simulink model "model_comp_19b"  (R2019b)
settings: Solver=ode45  StartTime=0.0  StopTime=100  RelTol=1e-3  EnableMultiTasking=on
values from neighbouring files (symbols this model uses):
  KDspd = 0    [time_validation.m]
  KIspd = 0    [time_validation.m]
  KPspd = 20    [time_validation.m]
  PARSa = [ ... (first row only)    [Q_ART_par.m]
  PARSu = zeros(Nu,5)    [Q_ART_par.m]
  TOTALMASS = sum (M,'all')    [Q_ART_par.m]
  v_ref = vconst    (= 5.55555555556)    [time_validation.m]
undefined symbols (not defined in the file or in its folder): axle_rate_limit, BRAKE, brake_lag, brake_rate, DRIVE, Lspd, Nspd, RW, Tb, Tst, Uspd
libraries: CarMaker4SL x72, simulink x2, TruckMaker4SL x1
(part 2 of 3)

== system model_comp_19b/truckmaker model/TruckMaker/IPG Vehicle/CarAndTrailer/Steering ==
  note: When replacing the entire steering system,
      | be sure to disable the IPG steering model by using the steering
      | model 'Model Manager off' in the vehicle GUI.
  Sync_In : Inport
  VhclCtrl.Steering : Inport  Port=2
  Bus Creator1 : BusCreator  Inputs=16
  Bus Creator2 : BusCreator  Inputs=5
  Demux : Demux  Outputs=21
      settings: DisplayOption=none
  Steering : S-Function  FunctionName=TM_Sfun  Parameters='Steering'  SFunctionDeploymentMode=off  EnableBusSupport=off
  Terminator : Terminator
  Sync_Out : Outport
  Steer.IF : Outport  Port=2
  wires:
  Demux/21 -> Bus Creator2/5  "Steering IF R Inert"
  Demux/20 -> Bus Creator2/4  "Steering IF R Frc"
  Demux/19 -> Bus Creator2/3  "Steering IF L Inert"
  Demux/18 -> Bus Creator2/2  "Steering IF L Frc"
  Demux/17 -> Bus Creator2/1  "Steering IF SteerByTrq"
  Demux/16 -> Bus Creator1/16  "Steering IF R iSteer2q"
  Demux/15 -> Bus Creator1/15  "Steering IF R qpp"
  Demux/14 -> Bus Creator1/14  "Steering IF R qp"
  Demux/13 -> Bus Creator1/13  "Steering IF R q"
  Demux/12 -> Bus Creator1/12  "Steering IF L iSteer2q"
  Demux/11 -> Bus Creator1/11  "Steering IF L qpp"
  Demux/10 -> Bus Creator1/10  "Steering IF L qp"
  Demux/9 -> Bus Creator1/9  "Steering IF L q"
  Demux/8 -> Bus Creator1/8  "Steering IF AssistTrqPin"
  Demux/7 -> Bus Creator1/7  "Steering IF AssistTrqCol"
  Demux/6 -> Bus Creator1/6  "Steering IF AssistFrc"
  Demux/5 -> Bus Creator1/5  "Steering IF TrqStatic"
  Demux/4 -> Bus Creator1/4  "Steering IF Trq"
  Demux/3 -> Bus Creator1/3  "Steering IF AngAcc"
  Demux/2 -> Bus Creator1/2  "Steering IF AngVel"
  Demux/1 -> Bus Creator1/1  "Steering IF Ang"
  Bus Creator1/1 -> Steer.IF/1
  Bus Creator2/1 -> Terminator/1  "Steer IF (in)"
  Sync_In/1 -> Steering/1
  Steering/1 -> Sync_Out/1
  VhclCtrl.Steering/1 -> Steering/2
  Steering/2 -> Demux/1

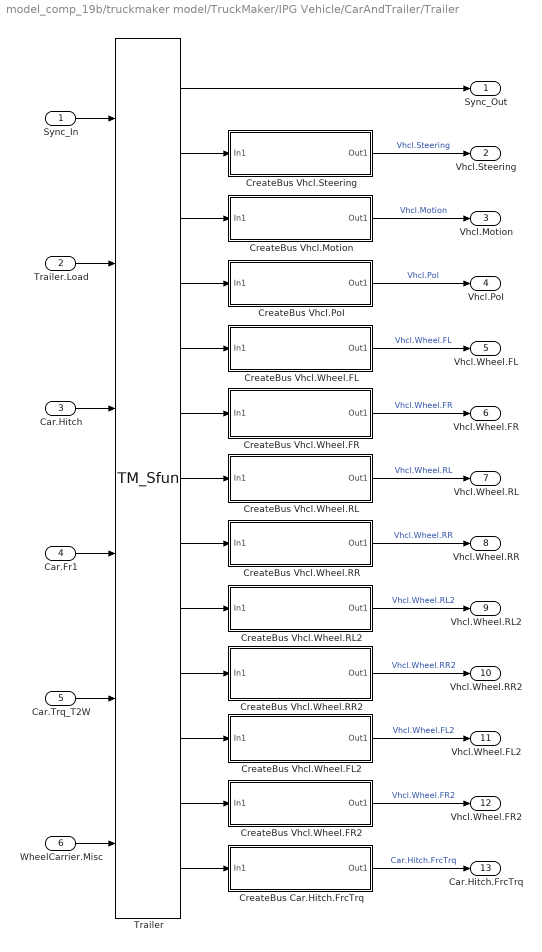
== system model_comp_19b/truckmaker model/TruckMaker/IPG Vehicle/CarAndTrailer/Trailer ==
  Sync_In : Inport
  Trailer.Load : Inport  Port=2
  Car.Hitch : Inport  Port=3
  Car.Fr1 : Inport  Port=4
  Car.Trq_T2W : Inport  Port=5
  WheelCarrier.Misc : Inport  Port=6
  CreateBus Car.Hitch.FrcTrq : Subsystem
  CreateBus Vhcl.Motion : Subsystem
  CreateBus Vhcl.PoI : Subsystem
  CreateBus Vhcl.Steering : Subsystem
  CreateBus Vhcl.Wheel.FL : Subsystem
  CreateBus Vhcl.Wheel.FL2 : Subsystem
  CreateBus Vhcl.Wheel.FR : Subsystem
  CreateBus Vhcl.Wheel.FR2 : Subsystem
  CreateBus Vhcl.Wheel.RL : Subsystem
  CreateBus Vhcl.Wheel.RL2 : Subsystem
  CreateBus Vhcl.Wheel.RR : Subsystem
  CreateBus Vhcl.Wheel.RR2 : Subsystem
  Trailer : S-Function  FunctionName=TM_Sfun  Parameters='Trailer'  SFunctionDeploymentMode=off  EnableBusSupport=off
  Sync_Out : Outport
  Vhcl.Steering : Outport  Port=2
  Vhcl.Motion : Outport  Port=3
  Vhcl.PoI : Outport  Port=4
  Vhcl.Wheel.FL : Outport  Port=5
  Vhcl.Wheel.FR : Outport  Port=6
  Vhcl.Wheel.RL : Outport  Port=7
  Vhcl.Wheel.RR : Outport  Port=8
  Vhcl.Wheel.RL2 : Outport  Port=9
  Vhcl.Wheel.RR2 : Outport  Port=10
  Vhcl.Wheel.FL2 : Outport  Port=11
  Vhcl.Wheel.FR2 : Outport  Port=12
  Car.Hitch.FrcTrq : Outport  Port=13
  wires:
  CreateBus Vhcl.Wheel.RL2/1(Out1) -> Vhcl.Wheel.RL2/1  "Vhcl.Wheel.RL2"
  CreateBus Vhcl.Wheel.RR2/1(Out1) -> Vhcl.Wheel.RR2/1  "Vhcl.Wheel.RR2"
  CreateBus Vhcl.Wheel.FL2/1(Out1) -> Vhcl.Wheel.FL2/1  "Vhcl.Wheel.FL2"
  CreateBus Vhcl.Wheel.FR2/1(Out1) -> Vhcl.Wheel.FR2/1  "Vhcl.Wheel.FR2"
  Trailer/12 -> CreateBus Vhcl.Wheel.FR2/1(In1)
  Trailer/11 -> CreateBus Vhcl.Wheel.FL2/1(In1)
  Trailer/10 -> CreateBus Vhcl.Wheel.RR2/1(In1)
  Trailer/9 -> CreateBus Vhcl.Wheel.RL2/1(In1)
  CreateBus Vhcl.Wheel.FL/1(Out1) -> Vhcl.Wheel.FL/1  "Vhcl.Wheel.FL"
  CreateBus Vhcl.Wheel.FR/1(Out1) -> Vhcl.Wheel.FR/1  "Vhcl.Wheel.FR"
  CreateBus Vhcl.Wheel.RL/1(Out1) -> Vhcl.Wheel.RL/1  "Vhcl.Wheel.RL"
  CreateBus Vhcl.Wheel.RR/1(Out1) -> Vhcl.Wheel.RR/1  "Vhcl.Wheel.RR"
  Trailer/8 -> CreateBus Vhcl.Wheel.RR/1(In1)
  Trailer/7 -> CreateBus Vhcl.Wheel.RL/1(In1)
  Trailer/6 -> CreateBus Vhcl.Wheel.FR/1(In1)
  Trailer/5 -> CreateBus Vhcl.Wheel.FL/1(In1)
  Trailer/13 -> CreateBus Car.Hitch.FrcTrq/1(In1)
  Trailer/2 -> CreateBus Vhcl.Steering/1(In1)
  CreateBus Vhcl.Steering/1(Out1) -> Vhcl.Steering/1  "Vhcl.Steering"
  Trailer/3 -> CreateBus Vhcl.Motion/1(In1)
  Trailer/4 -> CreateBus Vhcl.PoI/1(In1)
  CreateBus Vhcl.PoI/1(Out1) -> Vhcl.PoI/1  "Vhcl.PoI"
  CreateBus Vhcl.Motion/1(Out1) -> Vhcl.Motion/1  "Vhcl.Motion"
  Car.Trq_T2W/1 -> Trailer/5
  WheelCarrier.Misc/1 -> Trailer/6
  CreateBus Car.Hitch.FrcTrq/1(Out1) -> Car.Hitch.FrcTrq/1  "Car.Hitch.FrcTrq"
  Car.Fr1/1 -> Trailer/4
  Car.Hitch/1 -> Trailer/3
  Trailer.Load/1 -> Trailer/2
  Trailer/1 -> Sync_Out/1
  Sync_In/1 -> Trailer/1

== system model_comp_19b/truckmaker model/TruckMaker/IPG Vehicle/AFGc/brake and drive controller1/1&2 axle ==
  drive torque 1&2 : Inport
  Constant2 : Constant  Value=0
  Gain{,1..3} (4 alike) : Gain  Gain=-1
  Gain4 : Gain  Commented=through  Gain=-1
  To Workspace : ToWorkspace  VariableName=drive_torque1  SampleTime=-1
  Write CM Dict : CarMaker4SL/Write CM Dict  xname=PT.WFL.Trq_Drive  xsync=off
  Write CM Dict1 : CarMaker4SL/Write CM Dict  xname=PT.WFR.Trq_Drive  xsync=off
  Write CM Dict2 : CarMaker4SL/Write CM Dict  xname=PT.WRL.Trq_Drive  xsync=off
  Write CM Dict3 : CarMaker4SL/Write CM Dict  xname=PT.WRR.Trq_Drive  xsync=off
  Write CM Dict4 : CarMaker4SL/Write CM Dict  xname=PT.WFL.Trq_Supp2WC  xsync=off
  Write CM Dict5 : CarMaker4SL/Write CM Dict  xname=PT.WFR.Trq_Supp2WC  xsync=off
  Write CM Dict6 : CarMaker4SL/Write CM Dict  xname=PT.WRL.Trq_Supp2WC  xsync=off
  Write CM Dict7 : CarMaker4SL/Write CM Dict  xname=PT.WRR.Trq_Supp2WC  xsync=off
  Write CM Dict8 : CarMaker4SL/Write CM Dict  xname=PT.Trq_Supp2Bdy1B.y  xsync=off
  Write CM Dict9 : CarMaker4SL/Write CM Dict  xname=PT.Trq_Supp2Bdy1.y  xsync=off
  wires:
  Gain/1 -> Write CM Dict4/1
  Gain1/1 -> Write CM Dict5/1
  Gain2/1 -> Write CM Dict6/1
  Constant2/1 -> Write CM Dict8/1, Write CM Dict9/1
  drive torque 1&2/1 -> Gain4/1
  Gain3/1 -> Write CM Dict7/1
  Gain4/1 -> Gain/1, Write CM Dict/1, Gain1/1, Write CM Dict1/1, Write CM Dict2/1, Gain2/1, Gain3/1, Write CM Dict3/1, To Workspace/1

== system model_comp_19b/truckmaker model/TruckMaker/IPG Vehicle/AFGc/brake and drive controller1/7&8 axle ==
  drive torque 7&8 : Inport
  Gain4 : Gain  Commented=through  Gain=-1
  Terminator : Terminator  Commented=on
  To Workspace : ToWorkspace  VariableName=drive_torque7_8  SampleTime=-1
  Write CM Dict1 : CarMaker4SL/Write CM Dict  xname=Tr2.Trq_Ext2WhlML  xsync=off
  Write CM Dict2 : CarMaker4SL/Write CM Dict  xname=Tr2.Trq_Ext2WhlRL  xsync=off
  Write CM Dict3 : CarMaker4SL/Write CM Dict  xname=Tr2.Trq_Ext2WhlRR  xsync=off
  Write CM Dict4 : CarMaker4SL/Write CM Dict  xname=Tr2.Trq_Ext2WhlMR  xsync=off
  wires:
  drive torque 7&8/1 -> Gain4/1, To Workspace/1
  Gain4/1 -> Write CM Dict1/1, Write CM Dict4/1, Write CM Dict3/1, Write CM Dict2/1

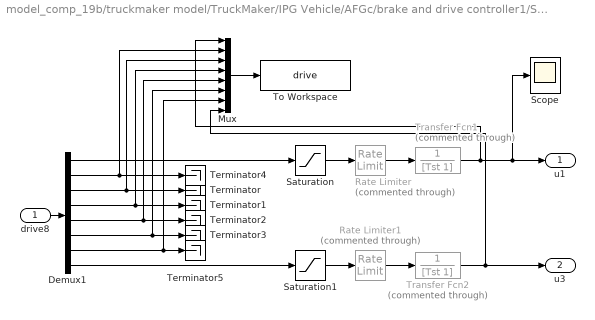
== system model_comp_19b/truckmaker model/TruckMaker/IPG Vehicle/AFGc/brake and drive controller1/Subsystem ==
  drive8 : Inport
  Demux1 : Demux  Outputs=8
  Mux : Mux  Inputs=8
  Rate Limiter : RateLimiter  Commented=through  RisingSlewLimit=500  FallingSlewLimit=-500  SampleTimeMode=inherited
  Rate Limiter1 : RateLimiter  Commented=through  RisingSlewLimit=500  FallingSlewLimit=-500  SampleTimeMode=inherited
  Saturation : Saturate  UpperLimit=1500  LowerLimit=0
  Saturation1 : Saturate  UpperLimit=1500  LowerLimit=0
  Scope : Scope
  Terminator{,1..5} (6 alike) : Terminator
  To Workspace : ToWorkspace  VariableName=drive  SampleTime=-1
  Transfer Fcn1 : TransferFcn  Commented=through  Denominator=[Tst 1]
  Transfer Fcn2 : TransferFcn  Commented=through  Denominator=[Tst 1]
  u1 : Outport
  u3 : Outport  Port=2
  wires:
  Demux1/3 -> Terminator/1, Mux/3
  Demux1/8 -> Saturation1/1
  Demux1/4 -> Terminator1/1, Mux/4
  drive8/1 -> Demux1/1
  Demux1/7 -> Terminator5/1, Mux/7
  Transfer Fcn2/1 -> Mux/8, u3/1
  Demux1/2 -> Mux/2, Terminator4/1
  Saturation1/1 -> Rate Limiter1/1
  Transfer Fcn1/1 -> Mux/1, Scope/1, u1/1
  Saturation/1 -> Rate Limiter/1
  Demux1/5 -> Terminator2/1, Mux/5
  Mux/1 -> To Workspace/1
  Demux1/6 -> Terminator3/1, Mux/6
  Demux1/1 -> Saturation/1
  Rate Limiter1/1 -> Transfer Fcn2/1
  Rate Limiter/1 -> Transfer Fcn1/1

== system model_comp_19b/truckmaker model/TruckMaker/IPG Vehicle/AFGc/brake and drive controller1/brakes ==
  note: torque reverses if wheel goes backwards
  brake torque command : Inport
  wheel speed : Inport  Port=2
  Memory : Memory
  Product : Product
  Rate Limiter : RateLimiter  RisingSlewLimit=brake_rate  FallingSlewLimit=-brake_rate  SampleTimeMode=inherited
  Sign : Signum
  Transport Delay : TransportDelay  Commented=on  DelayTime=brake_lag
  first_order_lags : Subsystem  Commented=on
  Out1 : Outport  VectorParamsAs1DForOutWhenUnconnected=off
  wires:
  Sign/1 -> Product/2
  Product/1 -> Out1/1
  Memory/1 -> Sign/1
  wheel speed/1 -> Memory/1
  Rate Limiter/1 -> Product/1
  Transport Delay/1 -> first_order_lags/1(In1)
  brake torque command/1 -> Rate Limiter/1

== system model_comp_19b/truckmaker model/TruckMaker/IPG Vehicle/AFGc/brake and drive controller1/brakes1 ==
  note: torque reverses if wheel goes backwards
  brake torque command : Inport
  wheel speed : Inport  Port=2
  Memory : Memory
  Product : Product
  Rate Limiter : RateLimiter  RisingSlewLimit=brake_rate  FallingSlewLimit=-brake_rate  SampleTimeMode=inherited
  Sign : Signum
  Transport Delay : TransportDelay  Commented=on  DelayTime=brake_lag
  first_order_lags : Subsystem  Commented=on
  Out1 : Outport  VectorParamsAs1DForOutWhenUnconnected=off
  wires:
  Sign/1 -> Product/2
  Product/1 -> Out1/1
  Memory/1 -> Sign/1
  wheel speed/1 -> Memory/1
  Rate Limiter/1 -> Product/1
  Transport Delay/1 -> first_order_lags/1(In1)
  brake torque command/1 -> Rate Limiter/1

== system model_comp_19b/truckmaker model/TruckMaker/IPG Vehicle/AFGc/brake and drive controller1/brakes2 ==
  note: torque reverses if wheel goes backwards
  brake torque command : Inport
  wheel speed : Inport  Port=2
  Memory : Memory
  Product : Product
  Rate Limiter : RateLimiter  RisingSlewLimit=brake_rate  FallingSlewLimit=-brake_rate  SampleTimeMode=inherited
  Sign : Signum
  Transport Delay : TransportDelay  Commented=on  DelayTime=brake_lag
  first_order_lags : Subsystem  Commented=on
  Out1 : Outport  VectorParamsAs1DForOutWhenUnconnected=off
  wires:
  Sign/1 -> Product/2
  Product/1 -> Out1/1
  Memory/1 -> Sign/1
  wheel speed/1 -> Memory/1
  Rate Limiter/1 -> Product/1
  Transport Delay/1 -> first_order_lags/1(In1)
  brake torque command/1 -> Rate Limiter/1

== system model_comp_19b/truckmaker model/TruckMaker/IPG Vehicle/AFGc/brake and drive controller1/passive torque distrubution ==
  note: convert to torque
  accel command : Inport
  BRAKE : Gain  Gain=BRAKE
  Constant : Constant  Value=0
  FWD : Gain  Gain=DRIVE
  Switch : Switch  Criteria=u2 > Threshold
  Switch1 : Switch  Criteria=u2 > Threshold
  "convert to 'total torque at the wheels\"" : Gain  Gain=TOTALMASS*RW  Multiplication=Matrix(K*u)
  drive torques : Outport  VectorParamsAs1DForOutWhenUnconnected=off
  brake torques : Outport  Port=2  VectorParamsAs1DForOutWhenUnconnected=off
  wires:
  accel command/1 -> "convert to 'total torque at the wheels\""/1
  Constant/1 -> Switch/3, Switch1/1
  Switch/1 -> FWD/1
  FWD/1 -> drive torques/1
  Switch1/1 -> BRAKE/1
  BRAKE/1 -> brake torques/1
  "convert to 'total torque at the wheels\""/1 -> Switch1/3, Switch1/2, Switch/1, Switch/2

== system model_comp_19b/truckmaker model/TruckMaker/IPG Vehicle/AFGc/brake and drive controller1/wheel speeds ==
  Mux1 : Mux  Inputs=3
  Read CM Dict1 : CarMaker4SL/Read CM Dict  xname=Car.WheelSpd_RL2  xsync=off  xstime=Continuous
  Read CM Dict10 : CarMaker4SL/Read CM Dict  xname=Car.WheelSpd_RL  xsync=off  xstime=Continuous
  Read CM Dict8 : CarMaker4SL/Read CM Dict  xname=Car.WheelSpd_FL  xsync=off  xstime=Continuous
  wheel speeds : Outport  VectorParamsAs1DForOutWhenUnconnected=off
  wires:
  Mux1/1 -> wheel speeds/1
  Read CM Dict1/1 -> Mux1/3
  Read CM Dict8/1 -> Mux1/1
  Read CM Dict10/1 -> Mux1/2

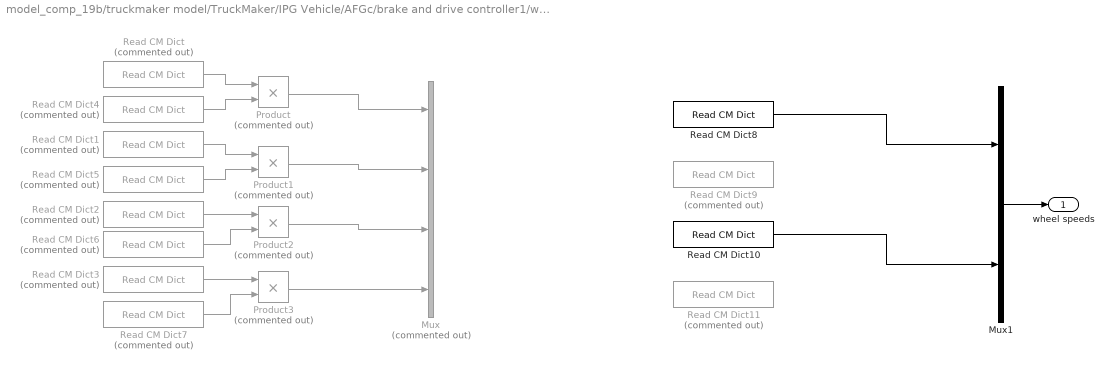
== system model_comp_19b/truckmaker model/TruckMaker/IPG Vehicle/AFGc/brake and drive controller1/wheel speeds1 ==
  Mux : Mux  Commented=on
  Mux1 : Mux  Inputs=2
  Product{,1..3} (4 alike) : Product  Commented=on
  Read CM Dict : CarMaker4SL/Read CM Dict  Commented=on  xname=Car.WheelSpd_FL  xsync=off  xstime=Continuous
  Read CM Dict1 : CarMaker4SL/Read CM Dict  Commented=on  xname=Car.WheelSpd_FR  xsync=off  xstime=Continuous
  Read CM Dict10 : CarMaker4SL/Read CM Dict  xname=Tr.WheelSpd_RL  xsync=off  xstime=Continuous
  Read CM Dict11 : CarMaker4SL/Read CM Dict  Commented=on  xname=Car.WheelSpd_RR  xsync=off  xstime=Continuous
  Read CM Dict2 : CarMaker4SL/Read CM Dict  Commented=on  xname=Car.WheelSpd_RL  xsync=off  xstime=Continuous
  Read CM Dict3 : CarMaker4SL/Read CM Dict  Commented=on  xname=Car.WheelSpd_RR  xsync=off  xstime=Continuous
  Read CM Dict4 : CarMaker4SL/Read CM Dict  Commented=on  xname=Car.WFL.Radius  xsync=off  xstime=Continuous
  Read CM Dict5 : CarMaker4SL/Read CM Dict  Commented=on  xname=Car.WFR.Radius  xsync=off  xstime=Continuous
  Read CM Dict6 : CarMaker4SL/Read CM Dict  Commented=on  xname=Car.WRL.Radius  xsync=off  xstime=Continuous
  Read CM Dict7 : CarMaker4SL/Read CM Dict  Commented=on  xname=Car.WRR.Radius  xsync=off  xstime=Continuous
  Read CM Dict8 : CarMaker4SL/Read CM Dict  xname=Tr.WheelSpd_FL  xsync=off  xstime=Continuous
  Read CM Dict9 : CarMaker4SL/Read CM Dict  Commented=on  xname=Car.WheelSpd_FR  xsync=off  xstime=Continuous
  wheel speeds : Outport  VectorParamsAs1DForOutWhenUnconnected=off
  wires:
  Read CM Dict/1 -> Product/1
  Read CM Dict4/1 -> Product/2
  Read CM Dict1/1 -> Product1/1
  Read CM Dict5/1 -> Product1/2
  Read CM Dict2/1 -> Product2/1
  Read CM Dict6/1 -> Product2/2
  Read CM Dict3/1 -> Product3/1
  Read CM Dict7/1 -> Product3/2
  Product/1 -> Mux/1
  Product1/1 -> Mux/2
  Product2/1 -> Mux/3
  Product3/1 -> Mux/4
  Mux1/1 -> wheel speeds/1
  Read CM Dict8/1 -> Mux1/1
  Read CM Dict10/1 -> Mux1/2

== system model_comp_19b/truckmaker model/TruckMaker/IPG Vehicle/AFGc/brake and drive controller1/wheel speeds2 ==
  Mux1 : Mux  Inputs=3
  Read CM Dict1 : CarMaker4SL/Read CM Dict  xname=Car.WheelSpd_RL  xsync=off  xstime=Continuous
  Read CM Dict10 : CarMaker4SL/Read CM Dict  xname=Car.WheelSpd_RL2  xsync=off  xstime=Continuous
  Read CM Dict8 : CarMaker4SL/Read CM Dict  xname=Car.WheelSpd_FL  xsync=off  xstime=Continuous
  wheel speeds : Outport  VectorParamsAs1DForOutWhenUnconnected=off
  wires:
  Mux1/1 -> wheel speeds/1
  Read CM Dict8/1 -> Mux1/1
  Read CM Dict10/1 -> Mux1/3
  Read CM Dict1/1 -> Mux1/2

== system model_comp_19b/truckmaker model/TruckMaker/IPG Vehicle/AFGc/q&qd builder/build q ==
  Read CM Dict : CarMaker4SL/Read CM Dict  xname=Tr.Yaw  xsync=off  xstime=Continuous
  Read CM Dict1 : CarMaker4SL/Read CM Dict  xname=Car.Yaw  xsync=off  xstime=Continuous
  Read CM Dict2 : CarMaker4SL/Read CM Dict  xname=Tr2.Yaw  xsync=off  xstime=Continuous
  Read CM Dict3 : CarMaker4SL/Read CM Dict  xname=Car.Fr1.tx  xsync=off  xstime=Continuous
  Read CM Dict5 : CarMaker4SL/Read CM Dict  xname=Car.Fr1.ty  xsync=off  xstime=Continuous
  generate q : MATLAB Function  TreatAsAtomicUnit=on
  q : Outport
  wires:
  Read CM Dict3/1 -> generate q/1(FR1x)
  Read CM Dict2/1 -> generate q/5(u3_yaw)
  Read CM Dict/1 -> generate q/4(u2_yaw)
  Read CM Dict1/1 -> generate q/3(u1_yaw)
  generate q/1(q) -> q/1
  Read CM Dict5/1 -> generate q/2(FR1y)

== system model_comp_19b/truckmaker model/TruckMaker/IPG Vehicle/AFGc/q&qd builder/build qd ==
  Read CM Dict1 : CarMaker4SL/Read CM Dict  xname=Car.Yaw  xsync=off  xstime=Continuous
  Read CM Dict2 : CarMaker4SL/Read CM Dict  xname=Tr.YawVel  xsync=off  xstime=Continuous
  Read CM Dict30 : CarMaker4SL/Read CM Dict  xname=Car.YawRate  xsync=off  xstime=Continuous
  Read CM Dict31 : CarMaker4SL/Read CM Dict  xname=Car.Fr1.vx  xsync=off  xstime=Continuous
  Read CM Dict32 : CarMaker4SL/Read CM Dict  xname=Car.Fr1.vy  xsync=off  xstime=Continuous
  Read CM Dict6 : CarMaker4SL/Read CM Dict  xname=Tr2.YawVel  xsync=off  xstime=Continuous
  generate qd : MATLAB Function  TreatAsAtomicUnit=on
  qd : Outport
  wires:
  Read CM Dict31/1 -> generate qd/1(vxFR1)
  Read CM Dict32/1 -> generate qd/2(vyFR1)
  Read CM Dict30/1 -> generate qd/3(u1_yaw_rate)
  Read CM Dict2/1 -> generate qd/4(u2_yaw_rate)
  Read CM Dict6/1 -> generate qd/5(u3_yaw_rate)
  Read CM Dict1/1 -> generate qd/6(u1_yaw_angle)
  generate qd/1(q_d) -> qd/1

== system model_comp_19b/truckmaker model/TruckMaker/IPG Vehicle/CarAndTrailer/CarAndTrailerUpd/CreateBus Brake.IF.In ==
  In : Inport
  BusCreator : BusCreator  Inputs=17
  Demux : Demux  Outputs=17
      settings: DisplayOption=none
  Out : Outport
  wires:
  Demux/17 -> BusCreator/17  "Brake IF Trq_Reg FR2"
  Demux/16 -> BusCreator/16  "Brake IF Trq_Reg FL2"
  Demux/15 -> BusCreator/15  "Brake IF Trq_Reg RR2"
  Demux/14 -> BusCreator/14  "Brake IF Trq_Reg RL2"
  Demux/13 -> BusCreator/13  "Brake IF Trq_Reg RR"
  Demux/12 -> BusCreator/12  "Brake IF Trq_Reg RL"
  Demux/11 -> BusCreator/11  "Brake IF Trq_Reg FR"
  Demux/10 -> BusCreator/10  "Brake IF Trq_Reg FL"
  Demux/9 -> BusCreator/9  "Brake IF Trq_Reg_max FR2"
  Demux/8 -> BusCreator/8  "Brake IF Trq_Reg_max FL2"
  Demux/7 -> BusCreator/7  "Brake IF Trq_Reg_max RR2"
  Demux/6 -> BusCreator/6  "Brake IF Trq_Reg_max RL2"
  Demux/5 -> BusCreator/5  "Brake IF Trq_Reg_max RR"
  Demux/4 -> BusCreator/4  "Brake IF Trq_Reg_max RL"
  Demux/3 -> BusCreator/3  "Brake IF Trq_Reg_max FR"
  Demux/2 -> BusCreator/2  "Brake IF Trq_Reg_max FL"
  Demux/1 -> BusCreator/1  "Brake IF T_env"
  BusCreator/1 -> Out/1
  In/1 -> Demux/1

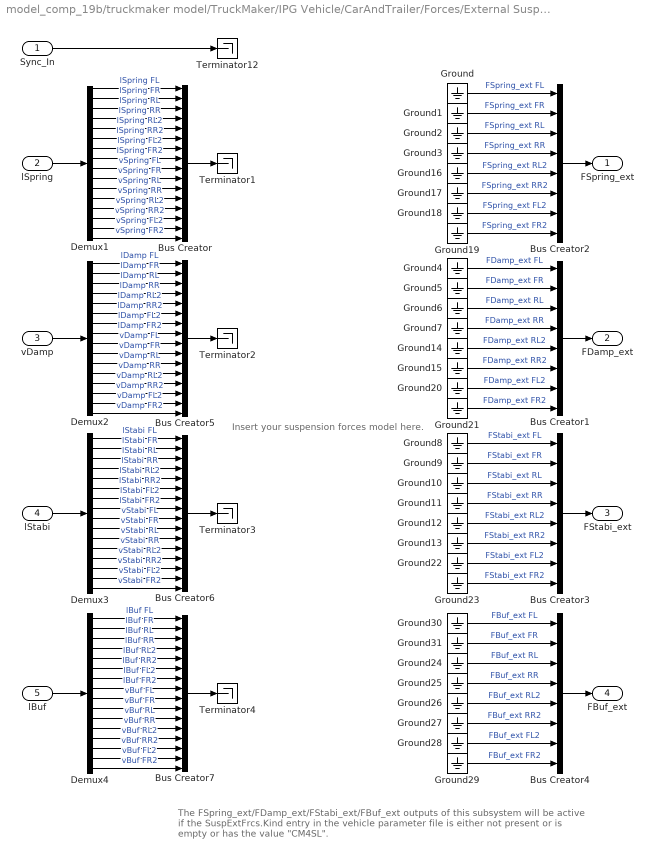
== system model_comp_19b/truckmaker model/TruckMaker/IPG Vehicle/CarAndTrailer/Forces/External Suspension Forces ==
  note: The FSpring_ext/FDamp_ext/FStabi_ext/FBuf_ext outputs of this subsystem will be
      | active if the SuspExtFrcs.Kind entry in the vehicle parameter file
      | is either not present or is empty or has the value "CM4SL".
  note: Insert your suspension forces model here.
  Sync_In : Inport
  lSpring : Inport  Port=2
  vDamp : Inport  Port=3
  lStabi : Inport  Port=4
  lBuf : Inport  Port=5
  Bus Creator{,5..7} (4 alike) : BusCreator  Inputs=16
  Bus Creator{1..4} (4 alike) : BusCreator  Inputs=8
  Demux{1..4} (4 alike) : Demux  Outputs=16
      settings: DisplayOption=none
  Ground{,1..31} (32 alike) : Ground
  Terminator{1..4,12} (5 alike) : Terminator
  FSpring_ext : Outport
  FDamp_ext : Outport  Port=2
  FStabi_ext : Outport  Port=3
  FBuf_ext : Outport  Port=4
  wires:
  Demux3/10 -> Bus Creator6/10  "vStabi FR"
  Demux4/16 -> Bus Creator7/16  "vBuf FR2"
  Demux4/15 -> Bus Creator7/15  "vBuf FL2"
  Demux4/14 -> Bus Creator7/14  "vBuf RR2"
  Demux4/13 -> Bus Creator7/13  "vBuf RL2"
  Demux4/12 -> Bus Creator7/12  "vBuf RR"
  Demux4/11 -> Bus Creator7/11  "vBuf RL"
  Demux4/10 -> Bus Creator7/10  "vBuf FR"
  Demux4/9 -> Bus Creator7/9  "vBuf FL"
  Demux3/16 -> Bus Creator6/16  "vStabi FR2"
  Demux3/15 -> Bus Creator6/15  "vStabi FL2"
  Demux3/14 -> Bus Creator6/14  "vStabi RR2"
  Demux3/13 -> Bus Creator6/13  "vStabi RL2"
  Demux3/12 -> Bus Creator6/12  "vStabi RR"
  Demux3/11 -> Bus Creator6/11  "vStabi RL"
  Demux3/9 -> Bus Creator6/9  "vStabi FL"
  Bus Creator6/1 -> Terminator3/1
  Bus Creator7/1 -> Terminator4/1
  Bus Creator5/1 -> Terminator2/1
  Bus Creator/1 -> Terminator1/1
  Demux2/16 -> Bus Creator5/16  "vDamp FR2"
  Demux2/15 -> Bus Creator5/15  "vDamp FL2"
  Demux2/14 -> Bus Creator5/14  "vDamp RR2"
  Demux2/13 -> Bus Creator5/13  "vDamp RL2"
  Demux2/12 -> Bus Creator5/12  "vDamp RR"
  Demux2/11 -> Bus Creator5/11  "vDamp RL"
  Demux2/10 -> Bus Creator5/10  "vDamp FR"
  Demux2/9 -> Bus Creator5/9  "vDamp FL"
  Demux1/16 -> Bus Creator/16  "vSpring FR2"
  Demux1/15 -> Bus Creator/15  "vSpring FL2"
  Demux1/14 -> Bus Creator/14  "vSpring RR2"
  Demux1/13 -> Bus Creator/13  "vSpring RL2"
  Demux1/12 -> Bus Creator/12  "vSpring RR"
  Demux1/11 -> Bus Creator/11  "vSpring RL"
  Demux1/10 -> Bus Creator/10  "vSpring FR"
  Demux1/9 -> Bus Creator/9  "vSpring FL"
  Demux3/7 -> Bus Creator6/7  "lStabi FL2"
  Demux3/8 -> Bus Creator6/8  "lStabi FR2"
  Ground22/1 -> Bus Creator3/7  "FStabi_ext FL2"
  Ground23/1 -> Bus Creator3/8  "FStabi_ext FR2"
  Demux2/7 -> Bus Creator5/7  "lDamp FL2"
  Demux2/8 -> Bus Creator5/8  "lDamp FR2"
  Ground20/1 -> Bus Creator1/7  "FDamp_ext FL2"
  Ground21/1 -> Bus Creator1/8  "FDamp_ext FR2"
  Ground18/1 -> Bus Creator2/7  "FSpring_ext FL2"
  Ground19/1 -> Bus Creator2/8  "FSpring_ext FR2"
  Demux1/7 -> Bus Creator/7  "lSpring FL2"
  Demux1/8 -> Bus Creator/8  "lSpring FR2"
  Sync_In/1 -> Terminator12/1
  lSpring/1 -> Demux1/1
  vDamp/1 -> Demux2/1
  lStabi/1 -> Demux3/1
  Demux3/1 -> Bus Creator6/1  "lStabi FL"
  Demux3/2 -> Bus Creator6/2  "lStabi FR"
  Demux3/3 -> Bus Creator6/3  "lStabi RL"
  Demux3/4 -> Bus Creator6/4  "lStabi RR"
  Demux1/1 -> Bus Creator/1  "lSpring FL"
  Demux1/2 -> Bus Creator/2  "lSpring FR"
  Demux1/3 -> Bus Creator/3  "lSpring RL"
  Demux1/4 -> Bus Creator/4  "lSpring RR"
  Demux2/1 -> Bus Creator5/1  "lDamp FL"
  Demux2/2 -> Bus Creator5/2  "lDamp FR"
  Demux2/3 -> Bus Creator5/3  "lDamp RL"
  Demux2/4 -> Bus Creator5/4  "lDamp RR"
  Bus Creator2/1 -> FSpring_ext/1
  Ground/1 -> Bus Creator2/1  "FSpring_ext FL"
  Ground1/1 -> Bus Creator2/2  "FSpring_ext FR"
  Ground2/1 -> Bus Creator2/3  "FSpring_ext RL"
  Ground3/1 -> Bus Creator2/4  "FSpring_ext RR"
  Ground4/1 -> Bus Creator1/1  "FDamp_ext FL"
  Ground5/1 -> Bus Creator1/2  "FDamp_ext FR"
  Ground6/1 -> Bus Creator1/3  "FDamp_ext RL"
  Ground7/1 -> Bus Creator1/4  "FDamp_ext RR"
  Bus Creator1/1 -> FDamp_ext/1
  Ground8/1 -> Bus Creator3/1  "FStabi_ext FL"
  Ground9/1 -> Bus Creator3/2  "FStabi_ext FR"
  Ground10/1 -> Bus Creator3/3  "FStabi_ext RL"
  Ground11/1 -> Bus Creator3/4  "FStabi_ext RR"
  Bus Creator3/1 -> FStabi_ext/1
  Demux3/5 -> Bus Creator6/5  "lStabi RL2"
  Demux3/6 -> Bus Creator6/6  "lStabi RR2"
  Ground12/1 -> Bus Creator3/5  "FStabi_ext RL2"
  Ground13/1 -> Bus Creator3/6  "FStabi_ext RR2"
  Demux2/5 -> Bus Creator5/5  "lDamp RL2"
  Demux2/6 -> Bus Creator5/6  "lDamp RR2"
  Ground14/1 -> Bus Creator1/5  "FDamp_ext RL2"
  Ground15/1 -> Bus Creator1/6  "FDamp_ext RR2"
  Demux1/5 -> Bus Creator/5  "lSpring RL2"
  Demux1/6 -> Bus Creator/6  "lSpring RR2"
  Ground16/1 -> Bus Creator2/5  "FSpring_ext RL2"
  Ground17/1 -> Bus Creator2/6  "FSpring_ext RR2"
  Demux4/7 -> Bus Creator7/7  "lBuf FL2"
  Demux4/8 -> Bus Creator7/8  "lBuf FR2"
  Ground28/1 -> Bus Creator4/7  "FBuf_ext FL2"
  Ground29/1 -> Bus Creator4/8  "FBuf_ext FR2"
  lBuf/1 -> Demux4/1
  Demux4/1 -> Bus Creator7/1  "lBuf FL"
  Demux4/2 -> Bus Creator7/2  "lBuf FR"
  Demux4/3 -> Bus Creator7/3  "lBuf RL"
  Demux4/4 -> Bus Creator7/4  "lBuf RR"
  Ground30/1 -> Bus Creator4/1  "FBuf_ext FL"
  Ground31/1 -> Bus Creator4/2  "FBuf_ext FR"
  Ground24/1 -> Bus Creator4/3  "FBuf_ext RL"
  Ground25/1 -> Bus Creator4/4  "FBuf_ext RR"
  Bus Creator4/1 -> FBuf_ext/1
  Demux4/5 -> Bus Creator7/5  "lBuf RL2"
  Demux4/6 -> Bus Creator7/6  "lBuf RR2"
  Ground26/1 -> Bus Creator4/5  "FBuf_ext RL2"
  Ground27/1 -> Bus Creator4/6  "FBuf_ext RR2"

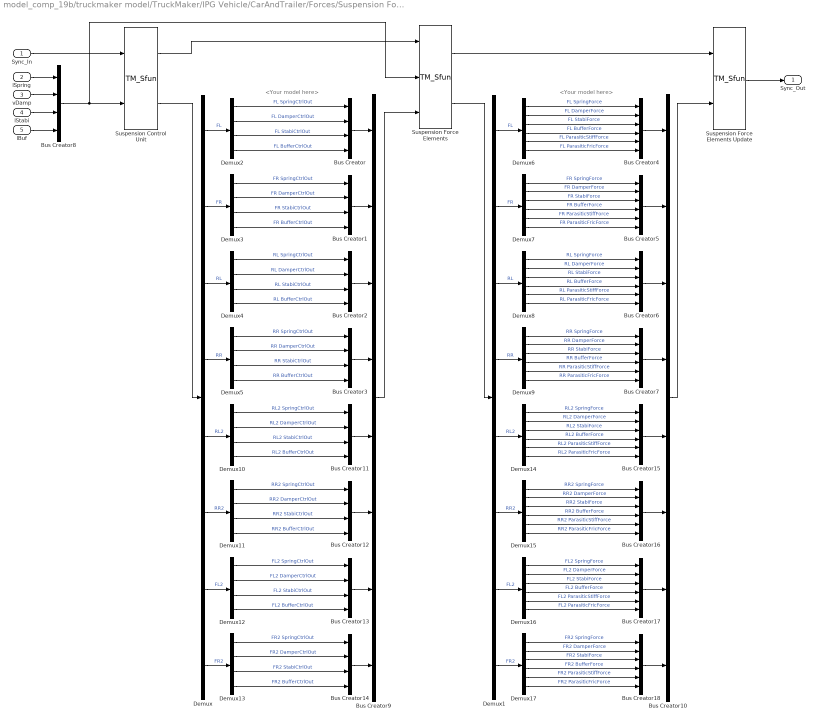
== system model_comp_19b/truckmaker model/TruckMaker/IPG Vehicle/CarAndTrailer/Forces/Suspension Forces ==
  note: <Your model here>
  note: <Your model here>
  Sync_In : Inport
  lSpring : Inport  Port=2
  vDamp : Inport  Port=3
  lStabi : Inport  Port=4
  lBuf : Inport  Port=5
  Bus Creator{,1..3,8,11..14} (9 alike) : BusCreator  Inputs=4
  Bus Creator10 : BusCreator  Inputs=8
  Bus Creator{4..7,15..18} (8 alike) : BusCreator  Inputs=6
  Bus Creator9 : BusCreator  Inputs=8
  Demux : Demux  Outputs=8
  Demux1 : Demux  Outputs=8
  Demux{2..5,10..13} (8 alike) : Demux
  Demux{6..9,14..17} (8 alike) : Demux  Outputs=6
  Suspension Control Unit : S-Function  FunctionName=TM_Sfun  Parameters='ForcesSuspControl'  SFunctionDeploymentMode=off  EnableBusSupport=off
  Suspension Force Elements : S-Function  FunctionName=TM_Sfun  Parameters='ForcesSusp'  SFunctionDeploymentMode=off  EnableBusSupport=off
  Suspension Force Elements Update : S-Function  FunctionName=TM_Sfun  Parameters='ForcesSuspUpd'  SFunctionDeploymentMode=off  EnableBusSupport=off
  Sync_Out : Outport
  wires:
  vDamp/1 -> Bus Creator8/2
  lStabi/1 -> Bus Creator8/3
  lBuf/1 -> Bus Creator8/4
  lSpring/1 -> Bus Creator8/1
  Bus Creator8/1 -> Suspension Control Unit/2, Suspension Force Elements/2
  Sync_In/1 -> Suspension Control Unit/1
  Suspension Control Unit/1 -> Suspension Force Elements/1
  Suspension Force Elements/1 -> Suspension Force Elements Update/1
  Suspension Force Elements Update/1 -> Sync_Out/1
  Bus Creator4/1 -> Bus Creator10/1
  Bus Creator5/1 -> Bus Creator10/2
  Bus Creator6/1 -> Bus Creator10/3
  Bus Creator7/1 -> Bus Creator10/4
  Demux6/1 -> Bus Creator4/1  "FL SpringForce"
  Demux9/1 -> Bus Creator7/1  "RR SpringForce"
  Demux9/2 -> Bus Creator7/2  "RR DamperForce"
  Demux9/3 -> Bus Creator7/3  "RR StabiForce"
  Demux9/4 -> Bus Creator7/4  "RR BufferForce"
  Demux9/5 -> Bus Creator7/5  "RR ParasiticStiffForce"
  Demux9/6 -> Bus Creator7/6  "RR ParasiticFricForce"
  Demux8/1 -> Bus Creator6/1  "RL SpringForce"
  Demux8/2 -> Bus Creator6/2  "RL DamperForce"
  Demux8/4 -> Bus Creator6/4  "RL BufferForce"
  Demux8/5 -> Bus Creator6/5  "RL ParasiticStiffForce"
  Demux8/6 -> Bus Creator6/6  "RL ParasiticFricForce"
  Demux8/3 -> Bus Creator6/3  "RL StabiForce"
  Demux7/1 -> Bus Creator5/1  "FR SpringForce"
  Demux7/2 -> Bus Creator5/2  "FR DamperForce"
  Demux7/3 -> Bus Creator5/3  "FR StabiForce"
  Demux7/4 -> Bus Creator5/4  "FR BufferForce"
  Demux7/5 -> Bus Creator5/5  "FR ParasiticStiffForce"
  Demux7/6 -> Bus Creator5/6  "FR ParasiticFricForce"
  Demux6/2 -> Bus Creator4/2  "FL DamperForce"
  Demux6/3 -> Bus Creator4/3  "FL StabiForce"
  Demux6/4 -> Bus Creator4/4  "FL BufferForce"
  Demux6/5 -> Bus Creator4/5  "FL ParasiticStiffForce"
  Demux6/6 -> Bus Creator4/6  "FL ParasiticFricForce"
  Bus Creator10/1 -> Suspension Force Elements Update/2
  Demux/1 -> Demux2/1  "FL"
  Bus Creator1/1 -> Bus Creator9/2
  Demux/2 -> Demux3/1  "FR"
  Bus Creator2/1 -> Bus Creator9/3
  Demux/3 -> Demux4/1  "RL"
  Bus Creator3/1 -> Bus Creator9/4
  Demux2/1 -> Bus Creator/1  "FL SpringCtrlOut"
  Demux/4 -> Demux5/1  "RR"
  Demux5/1 -> Bus Creator3/1  "RR SpringCtrlOut"
  Demux5/2 -> Bus Creator3/2  "RR DamperCtrlOut"
  Demux5/3 -> Bus Creator3/3  "RR StabiCtrlOut"
  Demux5/4 -> Bus Creator3/4  "RR BufferCtrlOut"
  Demux4/1 -> Bus Creator2/1  "RL SpringCtrlOut"
  Demux4/2 -> Bus Creator2/2  "RL DamperCtrlOut"
  Demux4/4 -> Bus Creator2/4  "RL BufferCtrlOut"
  Demux4/3 -> Bus Creator2/3  "RL StabiCtrlOut"
  Demux3/1 -> Bus Creator1/1  "FR SpringCtrlOut"
  Demux3/2 -> Bus Creator1/2  "FR DamperCtrlOut"
  Demux3/3 -> Bus Creator1/3  "FR StabiCtrlOut"
  Demux3/4 -> Bus Creator1/4  "FR BufferCtrlOut"
  Demux2/2 -> Bus Creator/2  "FL DamperCtrlOut"
  Demux2/3 -> Bus Creator/3  "FL StabiCtrlOut"
  Demux2/4 -> Bus Creator/4  "FL BufferCtrlOut"
  Suspension Control Unit/2 -> Demux/1
  Bus Creator9/1 -> Suspension Force Elements/3
  Bus Creator/1 -> Bus Creator9/1
  Suspension Force Elements/2 -> Demux1/1
  Demux1/1 -> Demux6/1  "FL"
  Demux1/2 -> Demux7/1  "FR"
  Demux1/3 -> Demux8/1  "RL"
  Demux1/4 -> Demux9/1  "RR"
  Demux/5 -> Demux10/1  "RL2"
  Bus Creator12/1 -> Bus Creator9/6
  Demux/6 -> Demux11/1  "RR2"
  Bus Creator13/1 -> Bus Creator9/7
  Demux/7 -> Demux12/1  "FL2"
  Bus Creator14/1 -> Bus Creator9/8
  Demux10/1 -> Bus Creator11/1  "RL2 SpringCtrlOut"
  Demux/8 -> Demux13/1  "FR2"
  Demux13/1 -> Bus Creator14/1  "FR2 SpringCtrlOut"
  Demux13/2 -> Bus Creator14/2  "FR2 DamperCtrlOut"
  Demux13/3 -> Bus Creator14/3  "FR2 StabiCtrlOut"
  Demux13/4 -> Bus Creator14/4  "FR2 BufferCtrlOut"
  Demux12/1 -> Bus Creator13/1  "FL2 SpringCtrlOut"
  Demux12/2 -> Bus Creator13/2  "FL2 DamperCtrlOut"
  Demux12/4 -> Bus Creator13/4  "FL2 BufferCtrlOut"
  Demux12/3 -> Bus Creator13/3  "FL2 StabiCtrlOut"
  Demux11/1 -> Bus Creator12/1  "RR2 SpringCtrlOut"
  Demux11/2 -> Bus Creator12/2  "RR2 DamperCtrlOut"
  Demux11/3 -> Bus Creator12/3  "RR2 StabiCtrlOut"
  Demux11/4 -> Bus Creator12/4  "RR2 BufferCtrlOut"
  Demux10/2 -> Bus Creator11/2  "RL2 DamperCtrlOut"
  Demux10/3 -> Bus Creator11/3  "RL2 StabiCtrlOut"
  Demux10/4 -> Bus Creator11/4  "RL2 BufferCtrlOut"
  Bus Creator11/1 -> Bus Creator9/5
  Bus Creator15/1 -> Bus Creator10/5
  Bus Creator16/1 -> Bus Creator10/6
  Bus Creator17/1 -> Bus Creator10/7
  Bus Creator18/1 -> Bus Creator10/8
  Demux14/1 -> Bus Creator15/1  "RL2 SpringForce"
  Demux17/1 -> Bus Creator18/1  "FR2 SpringForce"
  Demux17/2 -> Bus Creator18/2  "FR2 DamperForce"
  Demux17/3 -> Bus Creator18/3  "FR2 StabiForce"
  Demux17/4 -> Bus Creator18/4  "FR2 BufferForce"
  Demux17/5 -> Bus Creator18/5  "FR2 ParasiticStiffForce"
  Demux17/6 -> Bus Creator18/6  "FR2 ParasiticFricForce"
  Demux16/1 -> Bus Creator17/1  "FL2 SpringForce"
  Demux16/2 -> Bus Creator17/2  "FL2 DamperForce"
  Demux16/4 -> Bus Creator17/4  "FL2 BufferForce"
  Demux16/5 -> Bus Creator17/5  "FL2 ParasiticStiffForce"
  Demux16/6 -> Bus Creator17/6  "FL2 ParasiticFricForce"
  Demux16/3 -> Bus Creator17/3  "FL2 StabiForce"
  Demux15/1 -> Bus Creator16/1  "RR2 SpringForce"
  Demux15/2 -> Bus Creator16/2  "RR2 DamperForce"
  Demux15/3 -> Bus Creator16/3  "RR2 StabiForce"
  Demux15/4 -> Bus Creator16/4  "RR2 BufferForce"
  Demux15/5 -> Bus Creator16/5  "RR2 ParasiticStiffForce"
  Demux15/6 -> Bus Creator16/6  "RR2 ParasiticFricForce"
  Demux14/2 -> Bus Creator15/2  "RL2 DamperForce"
  Demux14/3 -> Bus Creator15/3  "RL2 StabiForce"
  Demux14/4 -> Bus Creator15/4  "RL2 BufferForce"
  Demux14/5 -> Bus Creator15/5  "RL2 ParasiticStiffForce"
  Demux14/6 -> Bus Creator15/6  "RL2 ParasiticFricForce"
  Demux1/5 -> Demux14/1  "RL2"
  Demux1/6 -> Demux15/1  "RR2"
  Demux1/7 -> Demux16/1  "FL2"
  Demux1/8 -> Demux17/1  "FR2"

== system model_comp_19b/truckmaker model/TruckMaker/IPG Vehicle/CarAndTrailer/Forces/Vehicle Forces ==
  Sync_In : Inport
  Bus Creator1 : BusCreator  Inputs=12
  Bus Creator8 : BusCreator  Inputs=16
  BusCreator1 : BusCreator  Inputs=4
  BusCreator2 : BusCreator  Inputs=9
  Demux : Demux  Outputs=16
      settings: DisplayOption=none
  Demux1 : Demux  Outputs=12
      settings: DisplayOption=none
  Demux2 : Demux  Outputs=13
      settings: DisplayOption=none
  Forces : S-Function  FunctionName=TM_Sfun  Parameters='Forces'  SFunctionDeploymentMode=off  EnableBusSupport=off
  Terminator : Terminator
  Sync_Out : Outport
  Car.Virtual : Outport  Port=2
  Car.Aero : Outport  Port=3
  Car.Load : Outport  Port=4
  wires:
  BusCreator1/1 -> Terminator/1  "Aero IF (in)"
  Demux2/13 -> BusCreator2/9  "car Aero Trq_1 z"
  Demux2/12 -> BusCreator2/8  "car Aero Trq_1 y"
  Demux2/11 -> BusCreator2/7  "car Aero Trq_1 x"
  Demux2/10 -> BusCreator2/6  "car Aero Frc_1 z"
  Demux2/9 -> BusCreator2/5  "car Aero Frc_1 y"
  Demux2/8 -> BusCreator2/4  "car Aero Frc_1 x"
  Demux2/7 -> BusCreator2/3  "car Aero PoA_1 z"
  Demux2/6 -> BusCreator2/2  "car Aero PoA_1 y"
  Demux2/5 -> BusCreator2/1  "car Aero PoA_1 x"
  Demux2/4 -> BusCreator1/4  "car Aero tau_1"
  Demux2/3 -> BusCreator1/3  "car Aero ApproachVel_1 z"
  Demux2/2 -> BusCreator1/2  "car Aero ApproachVel_1 y"
  Demux2/1 -> BusCreator1/1  "car Aero ApproachVel_1 x"
  BusCreator2/1 -> Car.Aero/1
  Demux/16 -> Bus Creator8/16  "Car Load_3 tz"
  Demux/15 -> Bus Creator8/15  "Car Load_3 ty"
  Demux/14 -> Bus Creator8/14  "Car Load_3 tx"
  Demux/13 -> Bus Creator8/13  "Car Load_3 mass"
  Demux1/12 -> Bus Creator1/12  "Car Virtual Trq_0 z"
  Demux1/11 -> Bus Creator1/11  "Car Virtual Trq_0 y"
  Demux1/10 -> Bus Creator1/10  "Car Virtual Trq_0 x"
  Demux1/9 -> Bus Creator1/9  "Car Virtual Trq_1 z"
  Demux1/8 -> Bus Creator1/8  "Car Virtual Trq_1 y"
  Demux1/7 -> Bus Creator1/7  "Car Virtual Trq_1 x"
  Demux1/6 -> Bus Creator1/6  "Car Virtual Frc_0 z"
  Demux1/5 -> Bus Creator1/5  "Car Virtual Frc_0 y"
  Demux1/4 -> Bus Creator1/4  "Car Virtual Frc_0 x"
  Sync_In/1 -> Forces/1
  Forces/1 -> Sync_Out/1
  Demux1/1 -> Bus Creator1/1  "Car Virtual Frc_1 x"
  Demux1/2 -> Bus Creator1/2  "Car Virtual Frc_1 y"
  Demux1/3 -> Bus Creator1/3  "Car Virtual Frc_1 z"
  Forces/3 -> Demux2/1
  Forces/2 -> Demux1/1
  Bus Creator1/1 -> Car.Virtual/1
  Bus Creator8/1 -> Car.Load/1
  Demux/1 -> Bus Creator8/1  "Car Load_0 mass"
  Demux/2 -> Bus Creator8/2  "Car Load_0 tx"
  Demux/3 -> Bus Creator8/3  "Car Load_0 ty"
  Demux/4 -> Bus Creator8/4  "Car Load_0 tz"
  Demux/5 -> Bus Creator8/5  "Car Load_1 mass"
  Demux/6 -> Bus Creator8/6  "Car Load_1 tx"
  Demux/7 -> Bus Creator8/7  "Car Load_1 ty"
  Demux/8 -> Bus Creator8/8  "Car Load_1 tz"
  Demux/9 -> Bus Creator8/9  "Car Load_2 mass"
  Demux/10 -> Bus Creator8/10  "Car Load_2 tx"
  Demux/11 -> Bus Creator8/11  "Car Load_2 ty"
  Demux/12 -> Bus Creator8/12  "Car Load_2 tz"
  Forces/4 -> Demux/1

== system model_comp_19b/truckmaker model/TruckMaker/IPG Vehicle/CarAndTrailer/Trailer/CreateBus Car.Hitch.FrcTrq ==
  In1 : Inport
  Bus Creator7 : BusCreator  Inputs=6
  Demux7 : Demux  Outputs=6
      settings: DisplayOption=none
  Out1 : Outport
  wires:
  In1/1 -> Demux7/1
  Bus Creator7/1 -> Out1/1
  Demux7/6 -> Bus Creator7/6  "Car Hitch Trq2Car z"
  Demux7/5 -> Bus Creator7/5  "Car Hitch Trq2Car y"
  Demux7/4 -> Bus Creator7/4  "Car Hitch Trq2Car x"
  Demux7/3 -> Bus Creator7/3  "Car Hitch Frc2Car z"
  Demux7/2 -> Bus Creator7/2  "Car Hitch Frc2Car y"
  Demux7/1 -> Bus Creator7/1  "Car Hitch Frc2Car x"

== system model_comp_19b/truckmaker model/TruckMaker/IPG Vehicle/CarAndTrailer/Trailer/CreateBus Vhcl.Motion ==
  In1 : Inport
  BusCreator : BusCreator  Inputs=15
  Demux : Demux  Outputs=15
      settings: DisplayOption=none
  Out1 : Outport
  wires:
  Demux/15 -> BusCreator/15  "Vhcl YawAcc"
  Demux/14 -> BusCreator/14  "Vhcl YawVel"
  Demux/13 -> BusCreator/13  "Vhcl Yaw"
  Demux/12 -> BusCreator/12  "Vhcl PitchAcc"
  Demux/11 -> BusCreator/11  "Vhcl PitchVel"
  Demux/10 -> BusCreator/10  "Vhcl Pitch"
  Demux/9 -> BusCreator/9  "Vhcl RollAcc"
  Demux/8 -> BusCreator/8  "Vhcl RollVel"
  Demux/7 -> BusCreator/7  "Vhcl Roll"
  Demux/6 -> BusCreator/6  "Vhcl Hitch_Pos z"
  Demux/5 -> BusCreator/5  "Vhcl Hitch_Pos y"
  Demux/4 -> BusCreator/4  "Vhcl Hitch_Pos x"
  Demux/3 -> BusCreator/3  "Vhcl sRoad"
  Demux/2 -> BusCreator/2  "Vhcl Distance"
  Demux/1 -> BusCreator/1  "Vhcl v"
  In1/1 -> Demux/1
  BusCreator/1 -> Out1/1

== system model_comp_19b/truckmaker model/TruckMaker/IPG Vehicle/CarAndTrailer/Trailer/CreateBus Vhcl.PoI ==
  In1 : Inport
  Bus Creator3 : BusCreator  Inputs=18
  Demux3 : Demux  Outputs=18
      settings: DisplayOption=none
  Out1 : Outport
  wires:
  Demux3/18 -> Bus Creator3/18  "Vhcl PoI_GCS Elev"
  Demux3/17 -> Bus Creator3/17  "Vhcl PoI_GCS Lat"
  Demux3/16 -> Bus Creator3/16  "Vhcl PoI_GCS Long"
  Demux3/15 -> Bus Creator3/15  "Vhcl PoI_Acc_1 z"
  Demux3/14 -> Bus Creator3/14  "Vhcl PoI_Acc_1 y"
  Demux3/13 -> Bus Creator3/13  "Vhcl PoI_Acc_1 x"
  Demux3/12 -> Bus Creator3/12  "Vhcl PoI_Vel_1 z"
  Demux3/11 -> Bus Creator3/11  "Vhcl PoI_Vel_1 y"
  Demux3/10 -> Bus Creator3/10  "Vhcl PoI_Vel_1 x"
  Demux3/9 -> Bus Creator3/9  "Vhcl PoI_Acc z"
  Demux3/8 -> Bus Creator3/8  "Vhcl PoI_Acc y"
  Demux3/7 -> Bus Creator3/7  "Vhcl PoI_Acc x"
  Demux3/6 -> Bus Creator3/6  "Vhcl PoI_Vel z"
  Demux3/5 -> Bus Creator3/5  "Vhcl PoI_Vel y"
  Demux3/4 -> Bus Creator3/4  "Vhcl PoI_Vel x"
  Demux3/3 -> Bus Creator3/3  "Vhcl PoI_Pos z"
  Demux3/2 -> Bus Creator3/2  "Vhcl PoI_Pos y"
  In1/1 -> Demux3/1
  Bus Creator3/1 -> Out1/1
  Demux3/1 -> Bus Creator3/1  "Vhcl PoI_Pos x"

== system model_comp_19b/truckmaker model/TruckMaker/IPG Vehicle/CarAndTrailer/Trailer/CreateBus Vhcl.Steering ==
  In1 : Inport
  Bus Creator3 : BusCreator  Inputs=4
  Demux : Demux
      settings: DisplayOption=none
  Out1 : Outport
  wires:
  Bus Creator3/1 -> Out1/1
  Demux/1 -> Bus Creator3/1  "Vhcl Steering Ang"
  Demux/3 -> Bus Creator3/3  "Vhcl Steering AngAcc"
  Demux/2 -> Bus Creator3/2  "Vhcl Steering AngVel"
  Demux/4 -> Bus Creator3/4  "Vhcl Steering Trq"
  In1/1 -> Demux/1

== system model_comp_19b/truckmaker model/TruckMaker/IPG Vehicle/CarAndTrailer/Trailer/CreateBus Vhcl.Wheel.FL ==
  In1 : Inport
  Bus Creator3 : BusCreator  Inputs=14
  Demux3 : Demux  Outputs=14
      settings: DisplayOption=none
  Out1 : Outport
  wires:
  Demux3/14 -> Bus Creator3/14  "Vhcl Wheel FL Trq_WhlBearing"
  Demux3/13 -> Bus Creator3/13  "Vhcl Wheel FL Trq_T2W"
  Demux3/12 -> Bus Creator3/12  "Vhcl Wheel FL SideSlip"
  Demux3/11 -> Bus Creator3/11  "Vhcl Wheel FL LongSlip"
  Demux3/10 -> Bus Creator3/10  "Vhcl Wheel FL vBelt"
  Demux3/9 -> Bus Creator3/9  "Vhcl Wheel FL Fz"
  Demux3/8 -> Bus Creator3/8  "Vhcl Wheel FL Fy"
  Demux3/7 -> Bus Creator3/7  "Vhcl Wheel FL Fx"
  Demux3/6 -> Bus Creator3/6  "Vhcl Wheel FL r_zxy z"
  Demux3/5 -> Bus Creator3/5  "Vhcl Wheel FL r_zxy y"
  Demux3/4 -> Bus Creator3/4  "Vhcl Wheel FL r_zxy x"
  Demux3/3 -> Bus Creator3/3  "Vhcl Wheel FL t z"
  Demux3/2 -> Bus Creator3/2  "Vhcl Wheel FL t y"
  In1/1 -> Demux3/1
  Bus Creator3/1 -> Out1/1
  Demux3/1 -> Bus Creator3/1  "Vhcl Wheel FL t x"

== system model_comp_19b/truckmaker model/TruckMaker/IPG Vehicle/CarAndTrailer/Trailer/CreateBus Vhcl.Wheel.FL2 ==
  In1 : Inport
  Bus Creator3 : BusCreator  Inputs=14
  Demux3 : Demux  Outputs=14
      settings: DisplayOption=none
  Out1 : Outport
  wires:
  Demux3/14 -> Bus Creator3/14  "Vhcl Wheel FL2 Trq_WhlBearing"
  Demux3/13 -> Bus Creator3/13  "Vhcl Wheel FL2 Trq_T2W"
  Demux3/12 -> Bus Creator3/12  "Vhcl Wheel FL2 SideSlip"
  Demux3/11 -> Bus Creator3/11  "Vhcl Wheel FL2 LongSlip"
  Demux3/10 -> Bus Creator3/10  "Vhcl Wheel FL2 vBelt"
  Demux3/9 -> Bus Creator3/9  "Vhcl Wheel FL2 Fz"
  Demux3/8 -> Bus Creator3/8  "Vhcl Wheel FL2 Fy"
  Demux3/7 -> Bus Creator3/7  "Vhcl Wheel FL2 Fx"
  Demux3/6 -> Bus Creator3/6  "Vhcl Wheel FL2 r_zxy z"
  Demux3/5 -> Bus Creator3/5  "Vhcl Wheel FL2 r_zxy y"
  Demux3/4 -> Bus Creator3/4  "Vhcl Wheel FL2 r_zxy x"
  Demux3/3 -> Bus Creator3/3  "Vhcl Wheel FL2 t z"
  Demux3/2 -> Bus Creator3/2  "Vhcl Wheel FL2 t y"
  In1/1 -> Demux3/1
  Bus Creator3/1 -> Out1/1
  Demux3/1 -> Bus Creator3/1  "Vhcl Wheel FL2 t x"

== system model_comp_19b/truckmaker model/TruckMaker/IPG Vehicle/CarAndTrailer/Trailer/CreateBus Vhcl.Wheel.FR ==
  In1 : Inport
  Bus Creator3 : BusCreator  Inputs=14
  Demux3 : Demux  Outputs=14
      settings: DisplayOption=none
  Out1 : Outport
  wires:
  Demux3/14 -> Bus Creator3/14  "Vhcl Wheel FR Trq_WhlBearing"
  Demux3/13 -> Bus Creator3/13  "Vhcl Wheel FR Trq_T2W"
  Demux3/12 -> Bus Creator3/12  "Vhcl Wheel FR SideSlip"
  Demux3/11 -> Bus Creator3/11  "Vhcl Wheel FR LongSlip"
  Demux3/10 -> Bus Creator3/10  "Vhcl Wheel FR vBelt"
  Demux3/9 -> Bus Creator3/9  "Vhcl Wheel FR Fz"
  Demux3/8 -> Bus Creator3/8  "Vhcl Wheel FR Fy"
  Demux3/7 -> Bus Creator3/7  "Vhcl Wheel FR Fx"
  Demux3/6 -> Bus Creator3/6  "Vhcl Wheel FR r_zxy z"
  Demux3/5 -> Bus Creator3/5  "Vhcl Wheel FR r_zxy y"
  Demux3/4 -> Bus Creator3/4  "Vhcl Wheel FR r_zxy x"
  Demux3/3 -> Bus Creator3/3  "Vhcl Wheel FR t z"
  Demux3/2 -> Bus Creator3/2  "Vhcl Wheel FR t y"
  In1/1 -> Demux3/1
  Bus Creator3/1 -> Out1/1
  Demux3/1 -> Bus Creator3/1  "Vhcl Wheel FR t x"

== system model_comp_19b/truckmaker model/TruckMaker/IPG Vehicle/CarAndTrailer/Trailer/CreateBus Vhcl.Wheel.FR2 ==
  In1 : Inport
  Bus Creator3 : BusCreator  Inputs=14
  Demux3 : Demux  Outputs=14
      settings: DisplayOption=none
  Out1 : Outport
  wires:
  Demux3/14 -> Bus Creator3/14  "Vhcl Wheel FR2 Trq_WhlBearing"
  Demux3/13 -> Bus Creator3/13  "Vhcl Wheel FR2 Trq_T2W"
  Demux3/12 -> Bus Creator3/12  "Vhcl Wheel FR2 SideSlip"
  Demux3/11 -> Bus Creator3/11  "Vhcl Wheel FR2 LongSlip"
  Demux3/10 -> Bus Creator3/10  "Vhcl Wheel FR2 vBelt"
  Demux3/9 -> Bus Creator3/9  "Vhcl Wheel FR2 Fz"
  Demux3/8 -> Bus Creator3/8  "Vhcl Wheel FR2 Fy"
  Demux3/7 -> Bus Creator3/7  "Vhcl Wheel FR2 Fx"
  Demux3/6 -> Bus Creator3/6  "Vhcl Wheel FR2 r_zxy z"
  Demux3/5 -> Bus Creator3/5  "Vhcl Wheel FR2 r_zxy y"
  Demux3/4 -> Bus Creator3/4  "Vhcl Wheel FR2 r_zxy x"
  Demux3/3 -> Bus Creator3/3  "Vhcl Wheel FR2 t z"
  Demux3/2 -> Bus Creator3/2  "Vhcl Wheel FR2 t y"
  In1/1 -> Demux3/1
  Bus Creator3/1 -> Out1/1
  Demux3/1 -> Bus Creator3/1  "Vhcl Wheel FR2 t x"

== system model_comp_19b/truckmaker model/TruckMaker/IPG Vehicle/CarAndTrailer/Trailer/CreateBus Vhcl.Wheel.RL ==
  In1 : Inport
  Bus Creator3 : BusCreator  Inputs=14
  Demux3 : Demux  Outputs=14
      settings: DisplayOption=none
  Out1 : Outport
  wires:
  Demux3/14 -> Bus Creator3/14  "Vhcl Wheel RL Trq_WhlBearing"
  Demux3/13 -> Bus Creator3/13  "Vhcl Wheel RL Trq_T2W"
  Demux3/12 -> Bus Creator3/12  "Vhcl Wheel RL SideSlip"
  Demux3/11 -> Bus Creator3/11  "Vhcl Wheel RL LongSlip"
  Demux3/10 -> Bus Creator3/10  "Vhcl Wheel RL vBelt"
  Demux3/9 -> Bus Creator3/9  "Vhcl Wheel RL Fz"
  Demux3/8 -> Bus Creator3/8  "Vhcl Wheel RL Fy"
  Demux3/7 -> Bus Creator3/7  "Vhcl Wheel RL Fx"
  Demux3/6 -> Bus Creator3/6  "Vhcl Wheel RL r_zxy z"
  Demux3/5 -> Bus Creator3/5  "Vhcl Wheel RL r_zxy y"
  Demux3/4 -> Bus Creator3/4  "Vhcl Wheel RL r_zxy x"
  Demux3/3 -> Bus Creator3/3  "Vhcl Wheel RL t z"
  Demux3/2 -> Bus Creator3/2  "Vhcl Wheel RL t y"
  In1/1 -> Demux3/1
  Bus Creator3/1 -> Out1/1
  Demux3/1 -> Bus Creator3/1  "Vhcl Wheel RL t x"

== system model_comp_19b/truckmaker model/TruckMaker/IPG Vehicle/CarAndTrailer/Trailer/CreateBus Vhcl.Wheel.RL2 ==
  In1 : Inport
  Bus Creator3 : BusCreator  Inputs=14
  Demux3 : Demux  Outputs=14
      settings: DisplayOption=none
  Out1 : Outport
  wires:
  Demux3/14 -> Bus Creator3/14  "Vhcl Wheel RL2 Trq_WhlBearing"
  Demux3/13 -> Bus Creator3/13  "Vhcl Wheel RL2 Trq_T2W"
  Demux3/12 -> Bus Creator3/12  "Vhcl Wheel RL2 SideSlip"
  Demux3/11 -> Bus Creator3/11  "Vhcl Wheel RL2 LongSlip"
  Demux3/10 -> Bus Creator3/10  "Vhcl Wheel RL2 vBelt"
  Demux3/9 -> Bus Creator3/9  "Vhcl Wheel RL2 Fz"
  Demux3/8 -> Bus Creator3/8  "Vhcl Wheel RL2 Fy"
  Demux3/7 -> Bus Creator3/7  "Vhcl Wheel RL2 Fx"
  Demux3/6 -> Bus Creator3/6  "Vhcl Wheel RL2 r_zxy z"
  Demux3/5 -> Bus Creator3/5  "Vhcl Wheel RL2 r_zxy y"
  Demux3/4 -> Bus Creator3/4  "Vhcl Wheel RL2 r_zxy x"
  Demux3/3 -> Bus Creator3/3  "Vhcl Wheel RL2 t z"
  Demux3/2 -> Bus Creator3/2  "Vhcl Wheel RL2 t y"
  In1/1 -> Demux3/1
  Bus Creator3/1 -> Out1/1
  Demux3/1 -> Bus Creator3/1  "Vhcl Wheel RL2 t x"

== system model_comp_19b/truckmaker model/TruckMaker/IPG Vehicle/CarAndTrailer/Trailer/CreateBus Vhcl.Wheel.RR ==
  In1 : Inport
  Bus Creator3 : BusCreator  Inputs=14
  Demux3 : Demux  Outputs=14
      settings: DisplayOption=none
  Out1 : Outport
  wires:
  Demux3/14 -> Bus Creator3/14  "Vhcl Wheel RR Trq_WhlBearing"
  Demux3/13 -> Bus Creator3/13  "Vhcl Wheel RR Trq_T2W"
  Demux3/12 -> Bus Creator3/12  "Vhcl Wheel RR SideSlip"
  Demux3/11 -> Bus Creator3/11  "Vhcl Wheel RR LongSlip"
  Demux3/10 -> Bus Creator3/10  "Vhcl Wheel RR vBelt"
  Demux3/9 -> Bus Creator3/9  "Vhcl Wheel RR Fz"
  Demux3/8 -> Bus Creator3/8  "Vhcl Wheel RR Fy"
  Demux3/7 -> Bus Creator3/7  "Vhcl Wheel RR Fx"
  Demux3/6 -> Bus Creator3/6  "Vhcl Wheel RR r_zxy z"
  Demux3/5 -> Bus Creator3/5  "Vhcl Wheel RR r_zxy y"
  Demux3/4 -> Bus Creator3/4  "Vhcl Wheel RR r_zxy x"
  Demux3/3 -> Bus Creator3/3  "Vhcl Wheel RR t z"
  Demux3/2 -> Bus Creator3/2  "Vhcl Wheel RR t y"
  In1/1 -> Demux3/1
  Bus Creator3/1 -> Out1/1
  Demux3/1 -> Bus Creator3/1  "Vhcl Wheel RR t x"

== system model_comp_19b/truckmaker model/TruckMaker/IPG Vehicle/CarAndTrailer/Trailer/CreateBus Vhcl.Wheel.RR2 ==
  In1 : Inport
  Bus Creator3 : BusCreator  Inputs=14
  Demux3 : Demux  Outputs=14
      settings: DisplayOption=none
  Out1 : Outport
  wires:
  Demux3/14 -> Bus Creator3/14  "Vhcl Wheel RR2 Trq_WhlBearing"
  Demux3/13 -> Bus Creator3/13  "Vhcl Wheel RR2 Trq_T2W"
  Demux3/12 -> Bus Creator3/12  "Vhcl Wheel RR2 SideSlip"
  Demux3/11 -> Bus Creator3/11  "Vhcl Wheel RR2 LongSlip"
  Demux3/10 -> Bus Creator3/10  "Vhcl Wheel RR2 vBelt"
  Demux3/9 -> Bus Creator3/9  "Vhcl Wheel RR2 Fz"
  Demux3/8 -> Bus Creator3/8  "Vhcl Wheel RR2 Fy"
  Demux3/7 -> Bus Creator3/7  "Vhcl Wheel RR2 Fx"
  Demux3/6 -> Bus Creator3/6  "Vhcl Wheel RR2 r_zxy z"
  Demux3/5 -> Bus Creator3/5  "Vhcl Wheel RR2 r_zxy y"
  Demux3/4 -> Bus Creator3/4  "Vhcl Wheel RR2 r_zxy x"
  Demux3/3 -> Bus Creator3/3  "Vhcl Wheel RR2 t z"
  Demux3/2 -> Bus Creator3/2  "Vhcl Wheel RR2 t y"
  In1/1 -> Demux3/1
  Bus Creator3/1 -> Out1/1
  Demux3/1 -> Bus Creator3/1  "Vhcl Wheel RR2 t x"

== system model_comp_19b/truckmaker model/TruckMaker/IPG Vehicle/AFGc/brake and drive controller1/brakes/first_order_lags ==
  In1 : Inport
  Demux : Demux  Outputs=2
      settings: DisplayOption=none
  Mux : Mux  Inputs=2
  Transfer Fcn : TransferFcn  Numerator=1  Denominator=[Tb 1]
  Transfer Fcn1 : TransferFcn  Numerator=1  Denominator=[Tb 1]
  Out1 : Outport  VectorParamsAs1DForOutWhenUnconnected=off
  wires:
  In1/1 -> Demux/1
  Mux/1 -> Out1/1
  Demux/1 -> Transfer Fcn/1
  Demux/2 -> Transfer Fcn1/1
  Transfer Fcn/1 -> Mux/1
  Transfer Fcn1/1 -> Mux/2

== system model_comp_19b/truckmaker model/TruckMaker/IPG Vehicle/AFGc/brake and drive controller1/brakes1/first_order_lags ==
  In1 : Inport
  Demux : Demux  Outputs=2
      settings: DisplayOption=none
  Mux : Mux  Inputs=2
  Transfer Fcn : TransferFcn  Numerator=1  Denominator=[Tb 1]
  Transfer Fcn1 : TransferFcn  Numerator=1  Denominator=[Tb 1]
  Out1 : Outport  VectorParamsAs1DForOutWhenUnconnected=off
  wires:
  In1/1 -> Demux/1
  Mux/1 -> Out1/1
  Demux/1 -> Transfer Fcn/1
  Demux/2 -> Transfer Fcn1/1
  Transfer Fcn/1 -> Mux/1
  Transfer Fcn1/1 -> Mux/2

== system model_comp_19b/truckmaker model/TruckMaker/IPG Vehicle/AFGc/brake and drive controller1/brakes2/first_order_lags ==
  In1 : Inport
  Demux : Demux  Outputs=2
      settings: DisplayOption=none
  Mux : Mux  Inputs=2
  Transfer Fcn : TransferFcn  Numerator=1  Denominator=[Tb 1]
  Transfer Fcn1 : TransferFcn  Numerator=1  Denominator=[Tb 1]
  Out1 : Outport  VectorParamsAs1DForOutWhenUnconnected=off
  wires:
  In1/1 -> Demux/1
  Mux/1 -> Out1/1
  Demux/1 -> Transfer Fcn/1
  Demux/2 -> Transfer Fcn1/1
  Transfer Fcn/1 -> Mux/1
  Transfer Fcn1/1 -> Mux/2

== matlab function model_comp_19b/truckmaker model/TruckMaker/IPG Vehicle/AFGc/q&qd builder/build q/generate q ==
  data: FR1x input; q output; FR1y input; u1_yaw input; u2_yaw input; u3_yaw input
function q =generate_q(FR1x,FR1y,u1_yaw,u2_yaw,u3_yaw)

l=11.4;%FR1 of u1 to front reference point


q=zeros(5,1);
q(1)=FR1x+l*cos(u1_yaw);
q(2)=FR1y+l*sin(u1_yaw);
q(3)=u1_yaw;
q(4)=u2_yaw;
q(5)=u3_yaw;
end

== matlab function model_comp_19b/truckmaker model/TruckMaker/IPG Vehicle/AFGc/MATLAB Function ==
  data: str1 input; y output; PARSa input
function y = StrMux(str1,PARSa)
%distribute steering from driver (and auto steer in future versions)
y=PARSa(:,6);
y=y*str1;
end

== matlab function model_comp_19b/truckmaker model/TruckMaker/IPG Vehicle/AFGc/find_vx1 ==
  settings: updateMethod=DISCRETE
  data: vx6 output; q input; qd input
function vx6 = vx_conversion(q,qd)
%#codegen
% convert q and qd to vx6 needed for the driver model

xxp=2; %nominal point P of driver 
u1=[cos(q(3));sin(q(3))];n1=[-sin(q(3));cos(q(3))];
rp = q(1:2)-xxp*u1;

v00=qd(1:2); %global velocity at front joint
vp=v00-qd(3)*xxp*n1; %move to driver point
U=dot(vp,u1);V=dot(vp,n1); %components in body axes (unit 1)
vx6=[U;V;qd(3);rp;q(3)]; %standard format ... [U,V,r,x,y,psi]'
end

== matlab function model_comp_19b/truckmaker model/TruckMaker/IPG Vehicle/AFGc/q&qd builder/build qd/generate qd ==
  data: vxFR1 input; q_d output; vyFR1 input; u1_yaw_rate input; u2_yaw_rate input; u3_yaw_rate input; u1_yaw_angle input
function q_d =generate_qd(vxFR1,vyFR1,u1_yaw_rate,u2_yaw_rate,u3_yaw_rate, u1_yaw_angle)

l=11.4;%FR1 of u1 to front reference point

q_d=zeros(5,1);

u1=[cos(u1_yaw_angle);sin(u1_yaw_angle)];n1=[-sin(u1_yaw_angle);cos(u1_yaw_angle)];

vfr1=[vxFR1;vyFR1];
q_d(1:2)=vfr1+u1_yaw_rate*l*n1;
% q_d(1)=vxFR1-l*u1_yaw_rate*cos(u1_yaw_angle);
% q_d(2)=vyFR1+l*u1_yaw_rate*sin(u1_yaw_angle);
q_d(3)=u1_yaw_rate;
q_d(4)=u2_yaw_rate;
q_d(5)=u3_yaw_rate;

end
